simulink model "cable_rob"  (R2023b)
settings: Solver=VariableStepAuto  StartTime=0.0  StopTime=simtime  RelTol=1e-3
values from neighbouring files (symbols this model uses):
  f_max = 100    [run.m]
  f_min = 10    [run.m]
  initialCondition = [y0;v0;l0']    [run.m]
  level = 2    [run.m]
  reference = [x_d; x_dd]    [run.m]
undefined symbols (not defined in the file or in its folder): a, b, Iz, mp
libraries: slpidlib x4
settings Model: Creator=aamo  LastModifiedBy=eliasoa

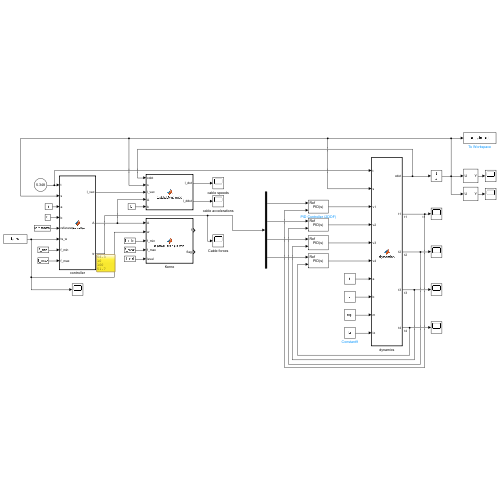
[thumbnail: Simulink's stored preview of the top-level diagram]
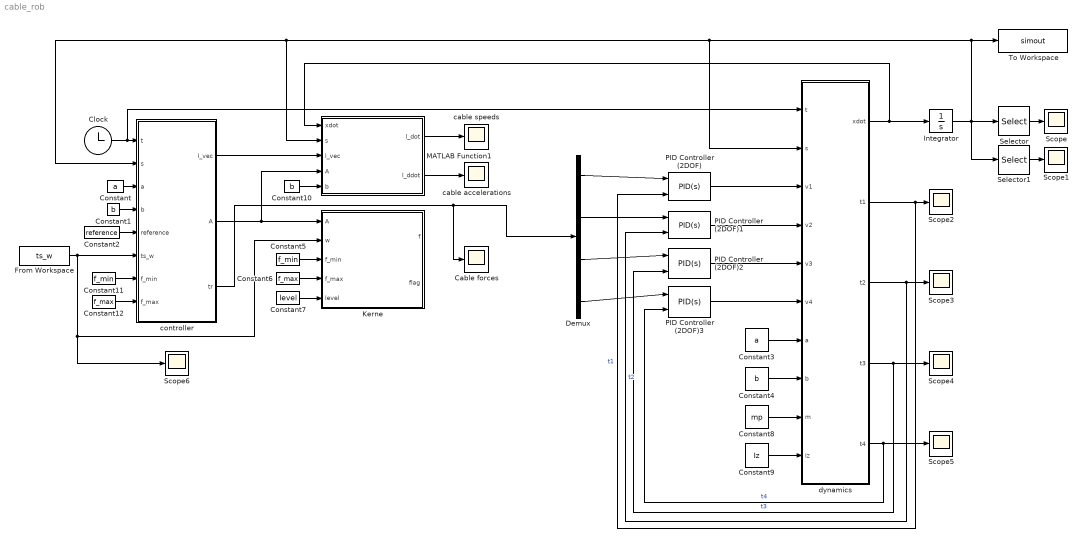
== system cable_rob ==
  Cable forces : Scope
  Clock : Clock
  Constant : Constant  Value=a
  Constant1 : Constant  Value=b
  Constant10 : Constant  Value=b
  Constant11 : Constant  Value=f_min
  Constant12 : Constant  Value=f_max
  Constant2 : Constant  Value=reference
  Constant3 : Constant  Value=a
  Constant4 : Constant  Value=b
  Constant5 : Constant  Value=f_min
  Constant6 : Constant  Value=f_max
  Constant7 : Constant  Value=level
  Constant8 : Constant  Value=mp
  Constant9 : Constant  Value=Iz
  Demux : Demux
  From Workspace : FromWorkspace  VariableName=ts_w  Interpolate=off  OutputAfterFinalValue=Setting to zero
  Integrator : Integrator  InitialCondition=initialCondition
  Kerne : MATLAB Function  TreatAsAtomicUnit=on
  MATLAB Function1 : MATLAB Function  TreatAsAtomicUnit=on
  PID Controller (2DOF){,1..3} (4 alike) : slpidlib/PID Controller (2DOF)  Controller=PID  Form=Parallel  TimeDomain=Continuous-time  UseExternalTs=off  SampleTime=-1  IntegratorMethod=Forward Euler  FilterMethod=Forward Euler  ControllerParametersSource=internal  P=10  I=1  UseKiTs=off  D=5  N=100  UseFilter=on  b=1  c=1  TunerSelectOption=Transfer Function Based (PID Tuner App)  InitialConditionSource=internal  InitialConditionForIntegrator=0  InitialConditionForFilter=0  DifferentiatorICPrevScaledInput=0  ExternalReset=none  TrackingMode=off  Kt=1  LimitOutput=off  SatLimitsSource=internal  UpperSaturationLimit=inf  LowerSaturationLimit=-inf  LinearizeAsGain=on  AntiWindupMode=none  Kb=1  LimitIntegrator=off  UpperIntegratorSaturationLimit=inf  LowerIntegratorSaturationLimit=-inf  POutMin=[]  POutMax=[]  IOutMin=[]  IOutMax=[]  DOutMin=[]  DOutMax=[]  NOutMin=[]  NOutMax=[]  bOutMin=[]  bOutMax=[]  cOutMin=[]  cOutMax=[]  SumOutMin=[]  SumOutMax=[]  SaturationOutMin=[]  SaturationOutMax=[]  PParamMin=[]  PParamMax=[]  IParamMin=[]  IParamMax=[]  DParamMin=[]  DParamMax=[]  NParamMin=[]  NParamMax=[]  bParamMin=[]  bParamMax=[]  cParamMin=[]  cParamMax=[]  KbParamMin=[]  KbParamMax=[]  KtParamMin=[]  KtParamMax=[]  KbOutMin=[]  KbOutMax=[]  KtOutMin=[]  KtOutMax=[]  IntegratorOutMin=[]  IntegratorOutMax=[]  FilterOutMin=[]  FilterOutMax=[]  SumI1OutMin=[]  SumI1OutMax=[]  SumI2OutMin=[]  SumI2OutMax=[]  SumI3OutMin=[]  SumI3OutMax=[]  SumI4OutMin=[]  SumI4OutMax=[]  SumDOutMin=[]  SumDOutMax=[]  Sum1OutMin=[]  Sum1OutMax=[]  Sum2OutMin=[]  Sum2OutMax=[]  Sum3OutMin=[]  Sum3OutMax=[]  DifferentiatorOutMin=[]  DifferentiatorOutMax=[]  FilterDiffOutCoefMin=[]  FilterDiffOutCoefMax=[]  ReciprocalOutMin=[]  ReciprocalOutMax=[]  SumDenOutMin=[]  SumDenOutMax=[]  SumNumOutMin=[]  SumNumOutMax=[]  DivideOutMin=[]  DivideOutMax=[]  UdiffTsProdOutMin=[]  UdiffTsProdOutMax=[]  NTsProdOutMin=[]  NTsProdOutMax=[]  UintegralTsProdOutMin=[]  UintegralTsProdOutMax=[]  UngainTsProdOutMin=[]  UngainTsProdOutMax=[]  ClampingZeroOutDataTypeStr=Inherit: Inherit via back propagation  ClampingZeroOutMin=[]  ClampingZeroOutMax=[]  FilterDenConstantOutDataTypeStr=Inherit: Inherit via back propagation  FilterDenConstantOutMin=[]  FilterDenConstantOutMax=[]  PCopyOutDataTypeStr=Inherit: Inherit via back propagation  PCopyOutMin=[]  PCopyOutMax=[]  NCopyOutDataTypeStr=Inherit: Inherit via back propagation  NCopyOutMin=[]  NCopyOutMax=[]  IntegratorContinuousStateAttributes=''  IntegratorStateMustResolveToSignalObject=off  IntegratorRTWStateStorageClass=Auto  FilterContinuousStateAttributes=''  FilterStateMustResolveToSignalObject=off  FilterRTWStateStorageClass=Auto  ParallelPVariant=InternalParameters  IdealPVariant=Disabled  IVariant=InternalParameters  DVariant=InternalParameters  bVariant=InternalParameters  cVariant=InternalParameters  IntegratorVariant=Continuous  SatVariant=Disabled  AWVariant=Passthrough  PCopyVariant=Disabled  TRVariant=Disabled  FdbkBlocksVariant=Forward  IdealPFdbkVariant=Disabled  SatFdbkVariant=Disabled  DerivativeFilterVariant=ContFilter  NVariant=InternalParameters  NCopyVariant=Disabled  FilterICVariant=InternalICsFilter  IntegratorICVariant=InternalICs  ExternalResetVariant=Disabled  TRSumVariant=Passthrough  SumFdbkVariant=Disabled  SumVariant=Sum_PID  TsampFilterVariant=InternalTs  TsampNgainVariant=Passthrough  TsampIntegralVariant=Disabled_SignalSpec  ExternalSaturationOutDataTypeStr=Inherit: Same as second input
  Scope{,1..6} (7 alike) : Scope
  Selector : Selector  InputPortWidth=10  IndexOptions=Index vector (dialog)  Indices=[1 2 3]  OutputSizes=1
  Selector1 : Selector  InputPortWidth=10  IndexOptions=Index vector (dialog)  Indices=[7 8 9 10]  OutputSizes=1
  To Workspace : ToWorkspace  VariableName=simout  SaveFormat=Timeseries  SampleTime=-1
  cable accelerations : Scope
  cable speeds : Scope
  controller : MATLAB Function  TreatAsAtomicUnit=on
  dynamics : MATLAB Function  TreatAsAtomicUnit=on
  wires:
  dynamics/1(xdot) -> Integrator/1, MATLAB Function1/1(xdot)
  Clock/1 -> dynamics/1(t), controller/1(t)
  Selector/1 -> Scope/1
  Selector1/1 -> Scope1/1
  PID Controller (2DOF)/1 -> dynamics/3(v1)
  PID Controller (2DOF)1/1 -> dynamics/4(v2)
  PID Controller (2DOF)2/1 -> dynamics/5(v3)
  PID Controller (2DOF)3/1 -> dynamics/6(v4)
  Constant/1 -> controller/3(a)
  Constant1/1 -> controller/4(b)
  Constant2/1 -> controller/5(reference)
  Constant4/1 -> dynamics/8(b)
  Constant3/1 -> dynamics/7(a)
  controller/2(A) -> MATLAB Function1/4(A), Kerne/1(A)
  Demux/1 -> PID Controller (2DOF)/1
  Demux/2 -> PID Controller (2DOF)1/1
  Demux/3 -> PID Controller (2DOF)2/1
  Demux/4 -> PID Controller (2DOF)3/1
  Constant8/1 -> dynamics/9(m)
  Constant9/1 -> dynamics/10(Iz)
  dynamics/3(t2) -> Scope3/1, PID Controller (2DOF)1/2  "t2"
  dynamics/4(t3) -> Scope4/1, PID Controller (2DOF)2/2  "t3"
  dynamics/5(t4) -> Scope5/1, PID Controller (2DOF)3/2  "t4"
  Constant10/1 -> MATLAB Function1/5(b)
  Integrator/1 -> dynamics/2(s), controller/2(s), MATLAB Function1/2(s), To Workspace/1, Selector/1, Selector1/1
  dynamics/2(t1) -> Scope2/1, PID Controller (2DOF)/2  "t1"
  MATLAB Function1/1(l_dot) -> cable speeds/1
  controller/1(l_vec) -> MATLAB Function1/3(l_vec)
  MATLAB Function1/2(l_ddot) -> cable accelerations/1
  From Workspace/1 -> Scope6/1, Kerne/2(w), controller/6(ts_w)
  Constant5/1 -> Kerne/3(f_min)
  Constant6/1 -> Kerne/4(f_max)
  Constant7/1 -> Kerne/5(level)
  Constant11/1 -> controller/7(f_min)
  Constant12/1 -> controller/8(f_max)
  controller/3(tr) -> Cable forces/1, Demux/1

== matlab function cable_rob/controller ==
  data: l_vec output; t input; A output; tr output; s input; a input; b input; reference input; ts_w input; f_min input; f_max input
function [l_vec,A,tr] = controller(t,s,a,b,reference,ts_w,f_min,f_max)
% Anchor points
a1 = a(:,1);
a2 = a(:,2);
a3 = a(:,3);
a4 = a(:,4);

% Position and rotation of actuator
% States
x = s(1); % x-position of actuator
y = s(2); % y-position of actuator
psi = s(3); % rotation of actuator

% Velocities
vx = s(4);
vy = s(5);
vr = s(6);

% Body anchors
b1 = b(:,1);
b2 = b(:,2);
b3 = b(:,3);
b4 = b(:,4);

% Body anchors in global coordinates
b1g = b_to_g([x;y],psi,b1);
b2g = b_to_g([x;y],psi,b2);
b3g = b_to_g([x;y],psi,b3);
b4g = b_to_g([x;y],psi,b4);

% Length of unstretched cable rolled out.
r1 = s(7);
r2 = s(8);
r3 = s(9);
r4 = s(10);

% % Compute tau.
% x_d = reference(1:3);
% x_dd = reference(4:6);
% 
% % x_d = 0.1*[sin(5*t);
% %        cos(5*t);
% %        0];
% % x_dd = 0.1*[5*cos(5*t);
% %         -5*sin(5*t);
% %         0];
% 
% 
% e = [x;y;psi]-x_d;
% e_d = [vx;vy;vr]-x_dd;
% D = 5*diag([1,1,1]);
% K = 7*diag([5,5,5]);
% tau_d = (-D*e_d-K*e);
% Compute tenstion setpoints.
%t1r = 20+5*sin(t/4+3);
%t2r = 20+5*sin(t/4+7);
%t3r = 20-5*sin(t/4+2);
%t4r = 20-5*sin(t/4+9);

% Cable vectors
l1_vec = (a1-b1g);
l2_vec = (a2-b2g);
l3_vec = (a3-b3g);
l4_vec = (a4-b4g);

l_vec = [l1_vec l2_vec l3_vec l4_vec];

% Compute force directions
Fd1 = l1_vec/norm(l1_vec);
Fd2 = l2_vec/norm(l2_vec);
Fd3 = l3_vec/norm(l3_vec);
Fd4 = l4_vec/norm(l4_vec);

% Compute resultant moment
R = [cos(psi), -sin(psi);sin(psi),cos(psi)];
M1 = cross([R*b1;0],[Fd1;0]);
M2 = cross([R*b2;0],[Fd2;0]);
M3 = cross([R*b3;0],[Fd3;0]);
M4 = cross([R*b4;0],[Fd4;0]);

A_transposed = [ Fd1,Fd2,Fd3,Fd4;
                 M1(3), M2(3), M3(3), M4(3)];

A = A_transposed';

coder.extrinsic('quadprog');
coder.extrinsic('optimoptions');
options = optimoptions('quadprog','Display','off');
tr = zeros(4,1);
tr = quadprog(eye(4),-10*ones(4,1),[],[],A_transposed, -ts_w,f_min*ones(4,1),f_max*ones(4,1), [], options);

% t1r = tr(1);
% t2r = tr(1);
% t3r = tr(1);
% t4r = tr(1);

== matlab function cable_rob/dynamics ==
  data: t input; xdot output; s input; t1 output; t2 output; t3 output; t4 output; v1 input; v2 input; v3 input; v4 input; a input; b input; m input; Iz input
function [xdot,t1,t2,t3,t4] = dynamics(t,s,v1,v2,v3,v4,a,b,m,Iz)

% Parameters
% m  Mass of actuator
% Iz Inertia of actuator

E=100E9;    % Young's modulus of wire
A= 1e-6;    % Cross sectional area of wire

% Anchor points
a1 = a(:,1);
a2 = a(:,2);
a3 = a(:,3);
a4 = a(:,4);

% Body anchors
b1 = b(:,1);
b2 = b(:,2);
b3 = b(:,3);
b4 = b(:,4);

% Position and rotation of actuator
% States
x = s(1); % x-position of actuator
y = s(2); % y-position of actuator
psi = s(3); % rotation of actuator

% Velocities
vx = s(4);
vy = s(5);
vr = s(6);

% Body anchors in global coordinates
b1g = b_to_g([x;y],psi,b1);
b2g = b_to_g([x;y],psi,b2);
b3g = b_to_g([x;y],psi,b3);
b4g = b_to_g([x;y],psi,b4);

% Length of unstretched cable rolled out.
r1 = s(7); 
r2 = s(8); 
r3 = s(9); 
r4 = s(10);

% Compute tensions.
t1 = A*E*(norm(b1g-a1) - r1) /r1;
t2 = A*E*(norm(b2g-a2) - r2) /r2;
t3 = A*E*(norm(b3g-a3) - r3) /r3;
t4 = A*E*(norm(b4g-a4) - r4) /r4;

% Compute forces
F1 = t1'*(a1-b1g)/norm(a1-b1g);
F2 = t2'*(a2-b2g)/norm(a2-b2g);
F3 = t3'*(a3-b3g)/norm(a3-b3g);
F4 = t4'*(a4-b4g)/norm(a4-b4g);

% Compute resultant force
F = F1+F2+F3+F4;

% Compute resultant moment
R = [cos(psi), -sin(psi);sin(psi),cos(psi)];
M1 = cross([R*b1;0],[F1;0]);
M2 = cross([R*b2;0],[F2;0]);
M3 = cross([R*b3;0],[F3;0]);
M4 = cross([R*b4;0],[F4;0]);

% Compute resultant moment
M = M1(3)+M2(3)+M3(3)+M4(3);

xdot = [vx;vy;vr;F(1)/m;F(2)/m;M/Iz;-v1;-v2;-v3;-v4];

% TESTING: direct feedthrough of desired tau.
% xdot = [vx;vy;vr;tau_d(1)/m;tau_d(2)/m;tau_d(3)/I;-v1;-v2;-v3;-v4];

== matlab function cable_rob/Kerne ==
  data: A input; f output; w input; f_min input; f_max input; level input; flag output
function [f, flag] = Kernel_translation(A,w,f_min,f_max,level)

[f, flag] = Kernel_translation(A,w,f_min,f_max,level);

== matlab function cable_rob/MATLAB Function1 ==
  data: xdot input; s input; l_dot output; l_vec input; A input; b input; l_ddot output
function [l_dot, l_ddot] = CableDynamics(xdot,s, l_vec,  A, b)
%   xdot:
%      u: matrix of the 4 cable unit vectors
% 

% Pose
x = s(1);
y = s(2);
psi = s(3);

% Velocities and accelerations of the platform
vx      = s(4);
vy      = s(5);
omega   = s(6);    % Angular Velocity
ax      = xdot(4);
ay      = xdot(5);
alpha   = xdot(6);    % Angular Acceleration

% Vector form
v_p     = [vx;vy];
omega_p = [0;0;omega];
a_p     = [ax;ay];
alpha_p = [0;0;alpha];

twist = [vx;vy;omega];

% Unstretched cable lengths
l = s(7:10);

% Dynamic Equation by Verhoeven

% 
% l_dot = zeros(4,1);
% for i = 1:4
%     b_dot = b_dot_g(v_p, omega_p, psi, b);
%     l_dot(i) = -[u(:,i), 0]'*b_dot;
% end

% Rate of change in cable lengths
l_dot = -A*twist; % Vector of absolute values

% Acceleration of change in cable lengths
l_ddot = zeros(4,1);

% Rotation Matrix
R = [cos(psi) -sin(psi);
     sin(psi) cos(psi)];

% Skew Symmetric Matrices to simplify cross-products
skew_omega = [0 -omega;omega 0];
skew_alpha = [0 -alpha;alpha 0];

for i = 1:4
    % Rate of change vector of cable length (3x1)
    l_i_dot = - v_p - skew_omega*R*b(:,i);

    % Unit cable vector
    u_i = l_vec(:,i)/norm(l_vec(:,i));
    
    % Derivative of unit cable vector
    u_i_dot = (l_i_dot*l(i) - l_vec(:,i) * l_dot(i)) * (1/l(i)^2);
    
    % Velocity of the point bi in inertial frame
    bi_dot = b_dot_g(v_p, omega, psi, b(:,i));

    % Acceleration of the point bi in inertial frame
    bi_ddot = a_p + skew_alpha*R*b(:,i)  +  skew_omega*skew_omega*R*b(:,i);


    % Acceleration of cable length
    l_ddot(i) = -u_i_dot'*bi_dot - u_i'*bi_ddot;
end
